simulink model "TheNotebookEdition_FeaturingAuto"  (R2024b)
settings: Solver=FixedStepAuto  StartTime=0.0  StopTime=inf  RelTol=1e-3  EnableMultiTasking=on
libraries: vexarmcortexlib x19, vexcommonlib x3
settings Model: Creator=ierdn  LastModifiedBy=vargi
settings DataIOCC: LimitDataPoints=on  SignalLoggingSaveFormat=ModelDataLogs  ReturnWorkspaceOutputs=off
settings OptimizationCC: ExpressionDepthLimit=2147483647  LifeSpan=Inf  MaxStackSize=64  EfficientTunableParamExpr=on
settings DebuggingCC: UnderspecifiedInitializationDetection=Classic  MergeDetectMultiDrivingBlocksExec=none  InheritedTsInSrcMsg=none  FcnCallInpInsideContextMsg=warning  StateNameClashWarn=warning  SFUnexpectedBacktrackingDiag=warning  SFNoUnconditionalDefaultTransitionDiag=warning  SFExecutionAtInitializationDiag=none  ArithmeticOperatorsInVariantConditions=warning
settings HardwareCC: ProdBitPerPointer=32  ProdBitPerSizeT=32  ProdBitPerPtrDiffT=32  ProdLargestAtomicInteger=Long  ProdLargestAtomicFloat=Double  ProdIntDivRoundTo=Undefined  ProdWordSize=32  ProdHWDeviceType=ARM Compatible->ARM Cortex
settings ModelReferenceCC: EnableRefExpFcnMdlSchedulingChecks=on  PropagateSignalLabelsOutOfModel=off
settings SFSimCC: MATLABDynamicMemAlloc=off  CustomCodeUndefinedFunction=UseInterfaceOnly
settings RTWCC: Description=Embedded Coder  SystemTargetFile=ert.tlc  HardwareBoard=ARM Cortex-based VEX Microcontroller  TemplateMakefile=ert_default_tmf  Toolchain=GNU Tools for VEX ARM Cortex  GPUComputeCapability=3.5
settings CodeAppCC: IgnoreCustomStorageClasses=off  CustomSymbolStrType=$N$R$M  StateflowObjectComments=on  InternalIdentifier=Classic
settings ERTTargetCC: CodeReplacementLibrary=GCC ARM Cortex-M3  MultiwordLength=2048  InlinedParameterPlacement=Hierarchical  ConvertIfToSwitch=off  SuppressUnreachableDefaultCases=off  DynamicArrayContainerType=coder::array

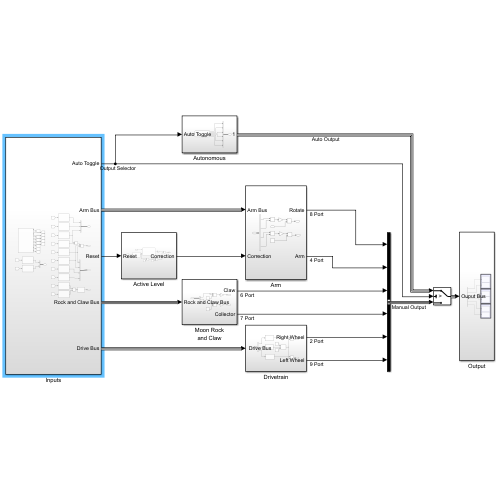
[thumbnail: Simulink's stored preview of the top-level diagram]
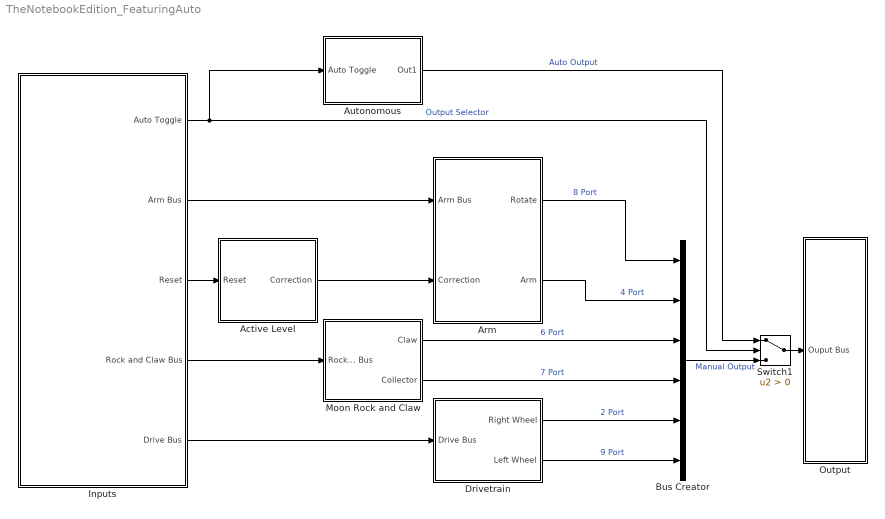
== system TheNotebookEdition_FeaturingAuto ==
  Active Level : Subsystem
  Arm : Subsystem
  Autonomous : Subsystem
  Bus Creator : BusCreator  Inputs=6
  Drivetrain : Subsystem
  Inputs : Subsystem
  Moon Rock and Claw : Subsystem
  Output : Subsystem
  Switch1 : Switch  Criteria=u2 > Threshold  SaturateOnIntegerOverflow=off  InputSameDT=off
  wires:
  Inputs/2(Arm Bus) -> Arm/1(Arm Bus)
  Inputs/4(Rock and Claw Bus) -> Moon Rock and Claw/1(Rock and Claw Bus)
  Inputs/3(Reset) -> Active Level/1(Reset)
  Inputs/5(" Drive Bus") -> Drivetrain/1(" Drive Bus")
  Active Level/1(Correction) -> Arm/2(Correction)
  Inputs/1(Auto Toggle) -> Autonomous/1(Auto Toggle), Switch1/2  "Output Selector"
  Arm/1(Rotate) -> Bus Creator/1  "8 Port"
  Arm/2(Arm) -> Bus Creator/2  "4 Port"
  Moon Rock and Claw/1(Claw) -> Bus Creator/3  "6 Port"
  Moon Rock and Claw/2(Collector) -> Bus Creator/4  "7 Port"
  Drivetrain/1(Right Wheel) -> Bus Creator/5  "2 Port"
  Drivetrain/2(Left Wheel) -> Bus Creator/6  "9 Port"
  Bus Creator/1 -> Switch1/3  "Manual Output"
  Switch1/1 -> Output/1(Ouput Bus)
  Autonomous/1(Out1) -> Switch1/1  "Auto Output"

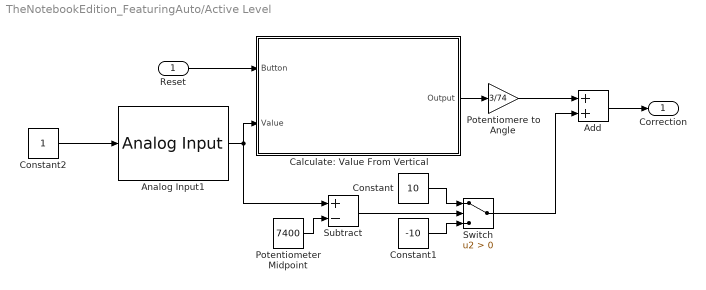
== system TheNotebookEdition_FeaturingAuto/Active Level ==
  Reset : Inport
  Add : Sum
  Analog Input1 : vexarmcortexlib/Sensors/Analog Input  inChan=1  SimulationIn=on  SampleTime=0.02
  Calculate: Value From Vertical : Stateflow chart  TreatAsAtomicUnit=on
  Constant : Constant  Value=10
  Constant1 : Constant  Value=-10
  Constant2 : Constant
  Potentiomere to Angle : Gain  Gain=3/74
  Potentiometer Midpoint : Constant  Value=7400
  Subtract : Sum  Inputs=+-
  Switch : Switch  Criteria=u2 > Threshold  SaturateOnIntegerOverflow=off  InputSameDT=off
  Correction : Outport
  wires:
  Calculate: Value From Vertical/1(Output) -> Potentiomere to Angle/1
  Analog Input1/1 -> Subtract/1, Calculate: Value From Vertical/2(Value)
  Reset/1 -> Calculate: Value From Vertical/1(Button)
  Constant/1 -> Switch/1
  Constant1/1 -> Switch/3
  Potentiomere to Angle/1 -> Add/1
  Switch/1 -> Add/2
  Add/1 -> Correction/1
  Constant2/1 -> Analog Input1/1
  Subtract/1 -> Switch/2
  Potentiometer Midpoint/1 -> Subtract/2

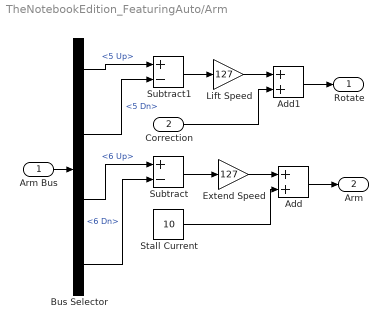
== system TheNotebookEdition_FeaturingAuto/Arm ==
  Arm Bus : Inport
  Correction : Inport  Port=2
  Add : Sum
  Add1 : Sum
  Bus Selector : BusSelector  OutputSignals=5 Up,5 Dn,6 Up,6 Dn
  Extend Speed : Gain  Gain=127
  Lift Speed : Gain  Gain=127
  Stall Current : Constant  Value=10
  Subtract : Sum  Inputs=+-
  Subtract1 : Sum  Inputs=+-
  Rotate : Outport
  Arm : Outport  Port=2
  wires:
  Bus Selector/1 -> Subtract1/1  "<5 Up>"
  Stall Current/1 -> Add/2
  Bus Selector/2 -> Subtract1/2  "<5 Dn>"
  Add/1 -> Arm/1
  Bus Selector/4 -> Subtract/2  "<6 Dn>"
  Bus Selector/3 -> Subtract/1  "<6 Up>"
  Arm Bus/1 -> Bus Selector/1
  Correction/1 -> Add1/2
  Add1/1 -> Rotate/1
  Subtract1/1 -> Lift Speed/1
  Lift Speed/1 -> Add1/1
  Subtract/1 -> Extend Speed/1
  Extend Speed/1 -> Add/1

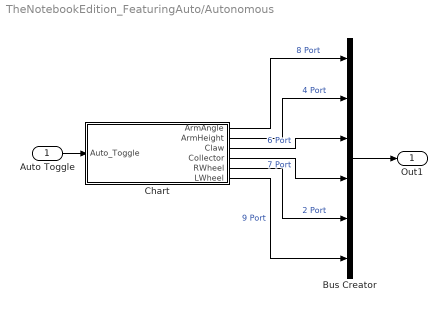
== system TheNotebookEdition_FeaturingAuto/Autonomous ==
  Auto Toggle : Inport
  Bus Creator : BusCreator  Inputs=6
  Chart : Stateflow chart  TreatAsAtomicUnit=on
  Out1 : Outport
  wires:
  Auto Toggle/1 -> Chart/1(Auto_Toggle)
  Bus Creator/1 -> Out1/1
  Chart/2(ArmHeight) -> Bus Creator/2  "4 Port"
  Chart/1(ArmAngle) -> Bus Creator/1  "8 Port"
  Chart/3(Claw) -> Bus Creator/3  "6 Port"
  Chart/4(Collector) -> Bus Creator/4  "7 Port"
  Chart/5(RWheel) -> Bus Creator/5  "2 Port"
  Chart/6(LWheel) -> Bus Creator/6  "9 Port"

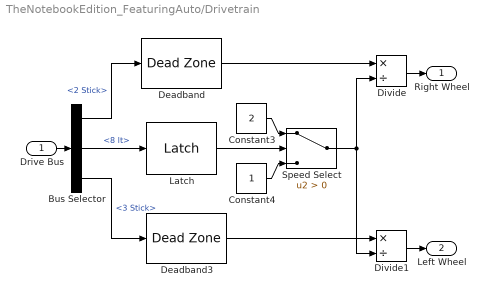
== system TheNotebookEdition_FeaturingAuto/Drivetrain ==
  " Drive Bus" : Inport
  Bus Selector : BusSelector  OutputSignals=2 Stick,8 lt,3 Stick
  Constant3 : Constant  Value=2
  Constant4 : Constant
  Deadband : DeadZone  LowerValue=-9  UpperValue=9
  Deadband3 : DeadZone  LowerValue=-9  UpperValue=9
  Divide : Product  Inputs=*/
  Divide1 : Product  Inputs=*/
  Latch : vexcommonlib/Latch  output0=off  BlockPlatform=vexarmcortex
  Speed Select : Switch  Criteria=u2 > Threshold  SaturateOnIntegerOverflow=off  InputSameDT=off
  Right Wheel : Outport
  Left Wheel : Outport  Port=2
  wires:
  Speed Select/1 -> Divide1/2, Divide/2
  Latch/1 -> Speed Select/2
  Constant3/1 -> Speed Select/1
  Deadband3/1 -> Divide1/1
  Constant4/1 -> Speed Select/3
  Deadband/1 -> Divide/1
  Divide/1 -> Right Wheel/1
  Divide1/1 -> Left Wheel/1
  " Drive Bus"/1 -> Bus Selector/1
  Bus Selector/1 -> Deadband/1  "<2 Stick>"
  Bus Selector/3 -> Deadband3/1  "<3 Stick>"
  Bus Selector/2 -> Latch/1  "<8 lt>"

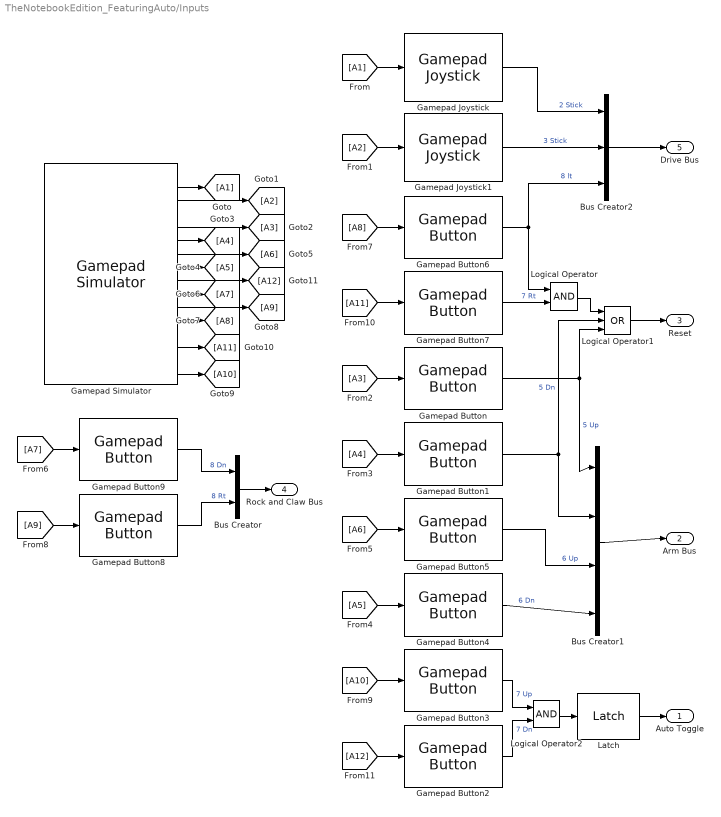
== system TheNotebookEdition_FeaturingAuto/Inputs ==
  Bus Creator : BusCreator  Inputs=2
  Bus Creator1 : BusCreator  Inputs=4
  Bus Creator2 : BusCreator  Inputs=3
  Gamepad Button : vexarmcortexlib/Gamepad/Gamepad Button  joystick=1  chan=5  button56=Up  button78=Down  SimulationIn=on  SampleTime=0.02
  Gamepad Button1 : vexarmcortexlib/Gamepad/Gamepad Button  joystick=1  chan=5  button56=Down  button78=Down  SimulationIn=on  SampleTime=0.02
  Gamepad Button2 : vexarmcortexlib/Gamepad/Gamepad Button  joystick=1  chan=8  button56=Up  button78=Up  SimulationIn=on  SampleTime=0.02
  Gamepad Button3 : vexarmcortexlib/Gamepad/Gamepad Button  joystick=1  chan=7  button56=Up  button78=Left  SimulationIn=on  SampleTime=0.02
  Gamepad Button4 : vexarmcortexlib/Gamepad/Gamepad Button  joystick=1  chan=6  button56=Down  button78=Down  SimulationIn=on  SampleTime=0.02
  Gamepad Button5 : vexarmcortexlib/Gamepad/Gamepad Button  joystick=1  chan=6  button56=Up  button78=Down  SimulationIn=on  SampleTime=0.02
  Gamepad Button6 : vexarmcortexlib/Gamepad/Gamepad Button  joystick=1  chan=8  button56=Up  button78=Left  SimulationIn=on  SampleTime=0.02
  Gamepad Button7 : vexarmcortexlib/Gamepad/Gamepad Button  joystick=1  chan=7  button56=Up  button78=Right  SimulationIn=on  SampleTime=0.02
  Gamepad Button8 : vexarmcortexlib/Gamepad/Gamepad Button  joystick=1  chan=8  button56=Up  button78=Right  SimulationIn=on  SampleTime=0.02
  Gamepad Button9 : vexarmcortexlib/Gamepad/Gamepad Button  joystick=1  chan=8  button56=Up  button78=Down  SimulationIn=on  SampleTime=0.02
  Gamepad Joystick : vexarmcortexlib/Gamepad/Gamepad Joystick  joystick=1  chan=2  SimulationIn=on  SampleTime=0.02
  Gamepad Joystick1 : vexarmcortexlib/Gamepad/Gamepad Joystick  joystick=1  chan=3  SimulationIn=on  SampleTime=0.02
  Gamepad Simulator : vexcommonlib/Gamepad Simulator  WhichPad=Logitech Gamepad  JoyId=1  BlockPlatform=vexarmcortex
      settings: LibrarySourceBlock=vexarmcortexlib/Utilities/Gamepad Simulator
  Latch : vexcommonlib/Latch  output0=off  BlockPlatform=vexarmcortex
      settings: LibrarySourceBlock=vexarmcortexlib/Utilities/Latch
  Logical Operator : Logic  AllPortsSameDT=off  OutDataTypeStr=boolean
  Logical Operator1 : Logic  Operator=OR  Inputs=3  AllPortsSameDT=off  OutDataTypeStr=boolean
  Logical Operator2 : Logic  AllPortsSameDT=off  OutDataTypeStr=boolean
  Auto Toggle : Outport
  Arm Bus : Outport  Port=2
  Reset : Outport  Port=3
  Rock and Claw Bus : Outport  Port=4
  " Drive Bus" : Outport  Port=5
  wires:
  Gamepad Button4/1 -> Bus Creator1/4  "6 Dn"
  Gamepad Button/1 -> Logical Operator1/3, Bus Creator1/1  "5 Up"
  Gamepad Button5/1 -> Bus Creator1/3  "6 Up"
  Gamepad Joystick/1 -> Bus Creator2/1  "2 Stick"
  Gamepad Joystick1/1 -> Bus Creator2/2  "3 Stick"
  Gamepad Button1/1 -> Logical Operator1/2, Bus Creator1/2  "5 Dn"
  Gamepad Button9/1 -> Bus Creator/1  "8 Dn"
  Gamepad Button8/1 -> Bus Creator/2  "8 Rt"
  Gamepad Button6/1 -> Logical Operator/1, Bus Creator2/3  "8 lt"
  Gamepad Button7/1 -> Logical Operator/2  "7 Rt"
  Bus Creator2/1 -> " Drive Bus"/1
  Logical Operator/1 -> Logical Operator1/1
  Bus Creator1/1 -> Arm Bus/1
  Bus Creator/1 -> Rock and Claw Bus/1
  Logical Operator1/1 -> Reset/1
  Gamepad Simulator/2 -> [A1]
  [A1] -> Gamepad Joystick/1
  Gamepad Simulator/3 -> [A2]
  [A2] -> Gamepad Joystick1/1
  Gamepad Simulator/5 -> [A3]
  [A3] -> Gamepad Button/1
  Gamepad Simulator/6 -> [A4]
  [A4] -> Gamepad Button1/1
  Gamepad Simulator/8 -> [A5]
  [A5] -> Gamepad Button4/1
  Gamepad Simulator/7 -> [A6]
  [A6] -> Gamepad Button5/1
  Gamepad Simulator/10 -> [A7]
  [A7] -> Gamepad Button9/1
  Gamepad Simulator/12 -> [A8]
  [A8] -> Gamepad Button6/1
  Gamepad Simulator/11 -> [A9]
  [A9] -> Gamepad Button8/1
  Gamepad Simulator/16 -> [A10]
  [A10] -> Gamepad Button3/1
  Gamepad Simulator/14 -> [A11]
  [A11] -> Gamepad Button7/1
  Gamepad Simulator/9 -> [A12]
  [A12] -> Gamepad Button2/1
  Gamepad Button3/1 -> Logical Operator2/1  "7 Up"
  Gamepad Button2/1 -> Logical Operator2/2  "7 Dn"
  Logical Operator2/1 -> Latch/1
  Latch/1 -> Auto Toggle/1

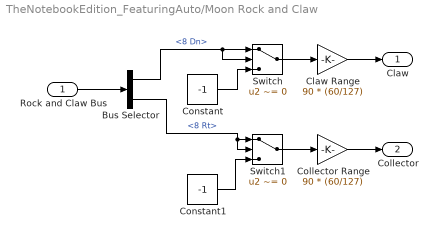
== system TheNotebookEdition_FeaturingAuto/Moon Rock and Claw ==
  Rock and Claw Bus : Inport
  Bus Selector : BusSelector  OutputSignals=8 Dn,8 Rt
  Claw Range : Gain  Gain=90 * (60/127)
  Collector Range : Gain  Gain=90 * (60/127)
  Constant : Constant  Value=-1
  Constant1 : Constant  Value=-1
  Switch : Switch  Criteria=u2 ~= 0  SaturateOnIntegerOverflow=off  InputSameDT=off
  Switch1 : Switch  Criteria=u2 ~= 0  SaturateOnIntegerOverflow=off  InputSameDT=off
  Claw : Outport
  Collector : Outport  Port=2
  wires:
  Switch1/1 -> Collector Range/1
  Bus Selector/2 -> Switch1/2, Switch1/1  "<8 Rt>"
  Collector Range/1 -> Collector/1
  Constant1/1 -> Switch1/3
  Claw Range/1 -> Claw/1
  Switch/1 -> Claw Range/1
  Constant/1 -> Switch/3
  Rock and Claw Bus/1 -> Bus Selector/1
  Bus Selector/1 -> Switch/2, Switch/1  "<8 Dn>"

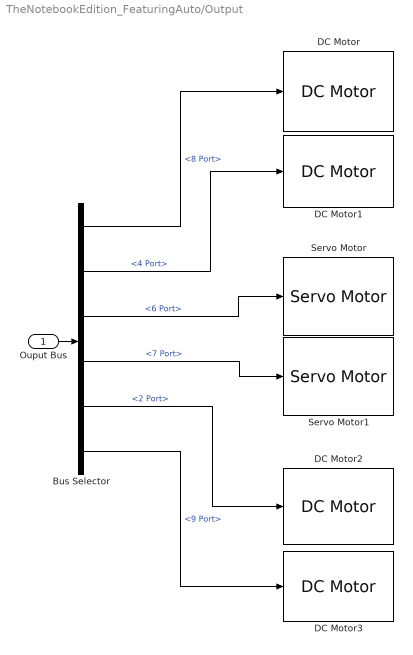
== system TheNotebookEdition_FeaturingAuto/Output ==
  Ouput Bus : Inport
  Bus Selector : BusSelector  OutputSignals=8 Port,4 Port,6 Port,7 Port,2 Port,9 Port
  DC Motor : vexarmcortexlib/Actuators/DC Motor  motor=8  scaleFactor=1/13.5  SimulationOut=off
  DC Motor1 : vexarmcortexlib/Actuators/DC Motor  motor=4  scaleFactor=1/13.5  SimulationOut=off
  DC Motor2 : vexarmcortexlib/Actuators/DC Motor  motor=2  scaleFactor=1/13.5  SimulationOut=off
  DC Motor3 : vexarmcortexlib/Actuators/DC Motor  motor=9  scaleFactor=1/13.5  SimulationOut=off
  Servo Motor : vexarmcortexlib/Actuators/Servo Motor  motor=6  scaleFactor=60/127  SimulationOut=off
  Servo Motor1 : vexarmcortexlib/Actuators/Servo Motor  motor=7  scaleFactor=60/127  SimulationOut=off
  wires:
  Ouput Bus/1 -> Bus Selector/1
  Bus Selector/1 -> DC Motor/1  "<8 Port>"
  Bus Selector/2 -> DC Motor1/1  "<4 Port>"
  Bus Selector/5 -> DC Motor2/1  "<2 Port>"
  Bus Selector/6 -> DC Motor3/1  "<9 Port>"
  Bus Selector/3 -> Servo Motor/1  "<6 Port>"
  Bus Selector/4 -> Servo Motor1/1  "<7 Port>"

== stateflow chart TheNotebookEdition_FeaturingAuto/Active Level/Calculate: Value From Vertical ==
  state Calculate
    Output = Value - Stored;
  state Start
    Stored = Value;
    Output = 0;
  (default) -> Start
  Start -> Calculate : [Button == 0]
  Calculate -> Start : [Button == 1]
  data: Output output; Stored local; Button input; Value input

== stateflow chart TheNotebookEdition_FeaturingAuto/Autonomous/Chart ==
  state Off
    LWheel = 0;
    RWheel = 0;
    Claw = -90;
    Collector = 0;
    ArmHeight = 0;
    ArmAngle = 0;
  state Approach
    LWheel = 50
    RWheel = 50
  state Grab
    LWheel = 0;
    RWheel = 0;
    Claw = 90;
  state Reverse
    LWheel = -50;
    RWheel = -50;
  (default) -> Off
  Reverse -> Off : [after(0.5,sec)]
  Off -> Approach : [Auto_Toggle == 1]
  Approach -> Grab : [after(0.5,sec)]
  Grab -> Reverse : [after(0.5,sec)]
  data: Auto_Toggle input; ArmAngle output; ArmHeight output; Claw output; Collector output; RWheel output; LWheel output
